simulink model "air_spring_zf"  (R2025a)
settings: Solver=VariableStepAuto  StartTime=0.0  StopTime=10.0  RelTol=1e-3
values from neighbouring files (symbols this model uses):
  c = 1500    [air_spring_script.m]
  k = 20000    [air_spring_script.m]
  m = 500    [air_spring_script.m]
settings Model: Creator=omrez  LastModifiedBy=omrez

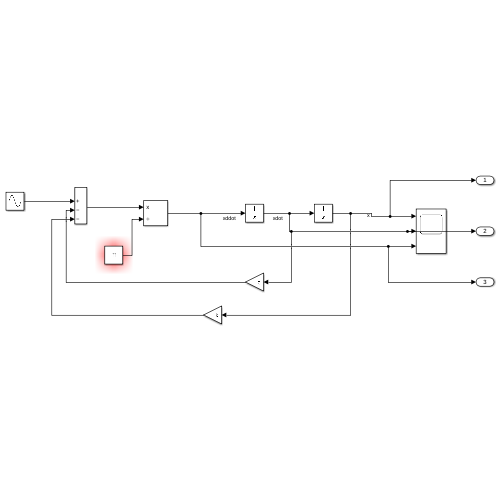
[thumbnail: Simulink's stored preview of the top-level diagram]
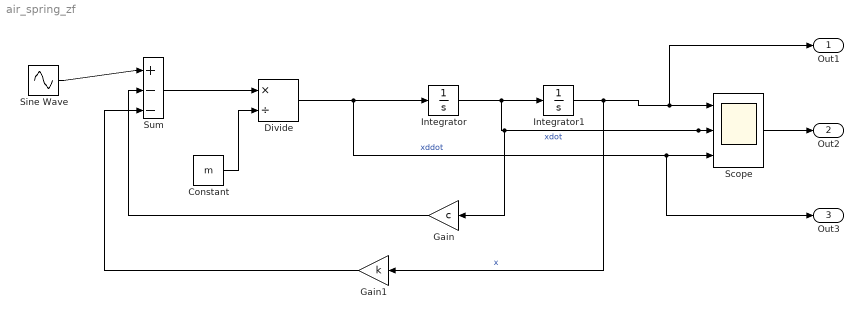
== system air_spring_zf ==
  Constant : Constant  Value=m
  Divide : Product  Inputs=*/
  Gain : Gain  Gain=c
  Gain1 : Gain  Gain=k
  Integrator : Integrator
  Integrator1 : Integrator
  Scope : Scope  NumInputPorts=3
  Sine Wave : Sin  Amplitude=15  Frequency=50  SampleTime=0
  Sum : Sum  Inputs=|+--
  Out1 : Outport
  Out2 : Outport  Port=2
  Out3 : Outport  Port=3
  wires:
  Sum/1 -> Divide/1
  Sine Wave/1 -> Sum/1
  Constant/1 -> Divide/2
  Divide/1 -> Out3/1, Scope/3, Integrator/1  "xddot"
  Integrator/1 -> Gain/1, Out2/1, Scope/2, Integrator1/1  "xdot"
  Integrator1/1 -> Gain1/1, Out1/1, Scope/1  "x"
  Gain/1 -> Sum/2
  Gain1/1 -> Sum/3
